simulink model "BD_EV"  (Simulink 7.9)
settings: Solver=ode1  SolverMode=SingleTasking  StartTime=0.0  StopTime=max(cyc_mph(:,1))  FixedStep=1  MaxStep=1  RelTol=1e-3  AbsTol=1e-3
libraries: lib_wheel x2, lib_help x2, lib_transmission x2, lib_outputs x1, lib_controls x1, lib_interactive x1, lib_drive_cycle x1, lib_accessory x1, lib_energy_storage x1, lib_electric_machine x1, lib_power_bus x1, lib_vehicle x1
settings Model: Creator=mokeefe  LastModifiedBy=mokeefe  ExtModeTrigMode=oneshot  ExtModeArmWhenConnect=off
settings Model: ModifiedComment=|
  | mokeefe -- Fri Mar 23 15:18:43 2012 -- Version 1.38
  | Updated parameterized link to restore library link. Save to update to newset Simulink version.
settings Model: ModifiedHistory=|
  | mokeefe -- Fri Mar 23 15:18:43 2012 -- Version 1.38
  | Updated parameterized link to restore library link. Save to update to newset Simulink version.
  | 
  | ssprik -- Wed Sep 24 14:52:29 2003 -- Version 1.37
  | 
  | 
  | abrooker -- Tue May 14 11:43:34 2002 -- Version 1.36
  | 
  | 
  | mokeefe -- Thu Apr 18 07:55:22 2002 -- Version 1.35
  | saving the model:
  | o "without the model browser open"
  | o with only top-level screen visible
  | o and with "fit to view" enabled
  | 
  | mokeefe -- Thu Apr 18 07:44:56 2002 -- Version 1.34
  | saving the model:
  | o "without the model browser open"
  | o with only top-level screen visible
  | o and with "fit to view" enabled
settings DataIOCC: LimitDataPoints=off  SaveOutput=off  SaveTime=off
settings OptimizationCC: BooleanDataType=off
settings DebuggingCC: SaveWithParameterizedLinksMsg=none  SignalResolutionControl=TryResolveAllWithWarning  SolverPrmCheckMsg=none  MultiTaskDSMMsg=warning  MultiTaskCondExecSysMsg=none  UnconnectedLineMsg=none  StrictBusMsg=None
settings HardwareCC: TargetUnknown=on
settings RTWCC: TemplateMakefile=grt_vc.tmf  IncludeERTFirstTime=on
settings GRTTargetCC: CombineOutputUpdateFcns=off  GRTInterface=on

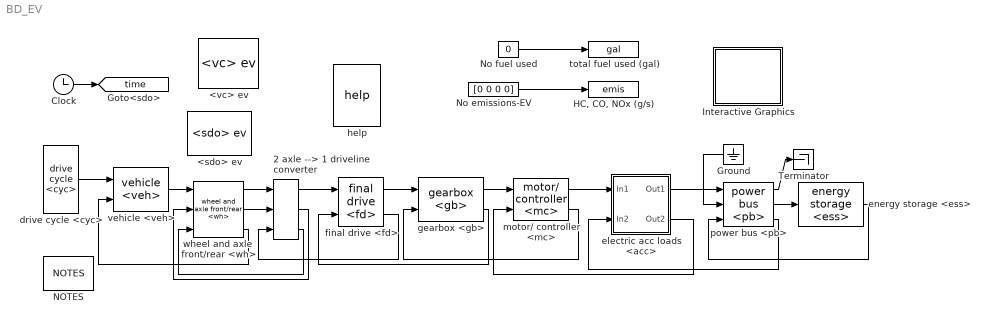
== system BD_EV ==
  2 axle --> 1 driveline converter : lib_wheel/2 axle --> 1 driveline converter
  <sdo> ev : lib_outputs/<sdo> ev  SystemSampleTime=-1
  <vc> ev : lib_controls/<vc> ev  SystemSampleTime=-1
  Clock : Clock
  Ground : Ground
  "HC, CO, NOx (g/s)" : ToWorkspace  VariableName=emis
  Interactive Graphics : Subsystem  BlockChoice=off
      settings: AttributesFormatString=%<BlockChoice>  TemplateBlock=lib_interactive/Interactive Graphics  MemberBlocks=off,on
  NOTES : lib_help/NOTES  SystemSampleTime=-1
  No emissions-EV : Constant  Value=[0 0 0 0]
  No fuel used : Constant  Value=0
  Terminator : Terminator
  drive cycle <cyc> : lib_drive_cycle/drive cycle <cyc>  SystemSampleTime=-1
  electric acc loads <acc> : Subsystem
      mask Display: image(imread('bdi_acc_elec.bmp'))
  energy storage <ess> : lib_energy_storage/energy storage <ess>  SystemSampleTime=-1
  final drive <fd> : lib_transmission/final drive <fd>  SystemSampleTime=-1
  gearbox <gb> : lib_transmission/gearbox <gb>  SystemSampleTime=-1
  help : lib_help/help  SystemSampleTime=-1
  motor/ controller <mc> : lib_electric_machine/motor// controller <mc>  SystemSampleTime=-1
  power bus <pb> : lib_power_bus/power bus <pb>  SystemSampleTime=-1
  total fuel used (gal) : ToWorkspace  VariableName=gal
  vehicle <veh> : lib_vehicle/vehicle <veh>  SystemSampleTime=-1
  wheel and axle  front/rear <wh> : lib_wheel/wheel and axle  front//rear <wh>  SystemSampleTime=-1
  tag scope: time=global
  wires:
  gearbox <gb>/1 -> motor/ controller <mc>/1
  final drive <fd>/2 -> 2 axle --> 1 driveline converter/3
  2 axle --> 1 driveline converter/1 -> final drive <fd>/1
  wheel and axle  front/rear <wh>/3 -> vehicle <veh>/2
  gearbox <gb>/2 -> final drive <fd>/2
  final drive <fd>/1 -> gearbox <gb>/1
  vehicle <veh>/1 -> wheel and axle  front/rear <wh>/1
  drive cycle <cyc>/1 -> vehicle <veh>/1
  Clock/1 -> [time]
  No fuel used/1 -> total fuel used (gal)/1
  No emissions-EV/1 -> "HC, CO, NOx (g/s)"/1
  motor/ controller <mc>/2 -> gearbox <gb>/2
  Ground/1 -> power bus <pb>/2
  energy storage <ess>/1 -> power bus <pb>/3
  power bus <pb>/2 -> energy storage <ess>/1
  power bus <pb>/1 -> Terminator/1
  motor/ controller <mc>/1 -> electric acc loads <acc>/1(In1)
  power bus <pb>/3 -> electric acc loads <acc>/2(In2)
  electric acc loads <acc>/1(Out1) -> power bus <pb>/1
  electric acc loads <acc>/2(Out2) -> motor/ controller <mc>/2
  wheel and axle  front/rear <wh>/1 -> 2 axle --> 1 driveline converter/1
  wheel and axle  front/rear <wh>/2 -> 2 axle --> 1 driveline converter/2
  2 axle --> 1 driveline converter/2 -> wheel and axle  front/rear <wh>/2
  2 axle --> 1 driveline converter/3 -> wheel and axle  front/rear <wh>/3

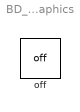
== system BD_EV/Interactive Graphics ==
  off : lib_interactive/off  Tag=Altia_off  SystemSampleTime=-1

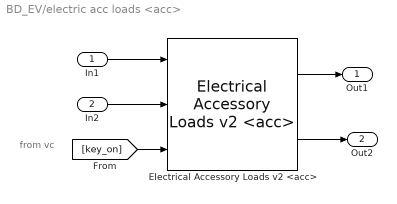
== system BD_EV/electric acc loads <acc> ==
  note: from vc
  In1 : Inport
  In2 : Inport  Port=2
  Electrical Accessory Loads v2 <acc> : lib_accessory/Electrical Accessory Loads v2 <acc>  load_on=1
  Out1 : Outport
  Out2 : Outport  Port=2
  wires:
  In1/1 -> Electrical Accessory Loads v2 <acc>/1
  In2/1 -> Electrical Accessory Loads v2 <acc>/2
  Electrical Accessory Loads v2 <acc>/1 -> Out1/1
  Electrical Accessory Loads v2 <acc>/2 -> Out2/1
  [key_on] -> Electrical Accessory Loads v2 <acc>/3
